simulink model "testBP"  (R2023a)
settings: Solver=VariableStepAuto  StartTime=0.0  StopTime=10.0  RelTol=1e-3
settings Model: Creator=grouleau  LastModifiedBy=grouleau
settings OptimizationCC: AccelVerboseBuild=on
settings SFSimCC: SimCustomHeaderCode="#include \"myFunc.h\""  SimUserSources=myFunc.c  SimDebugExecutionForCustomCode=on

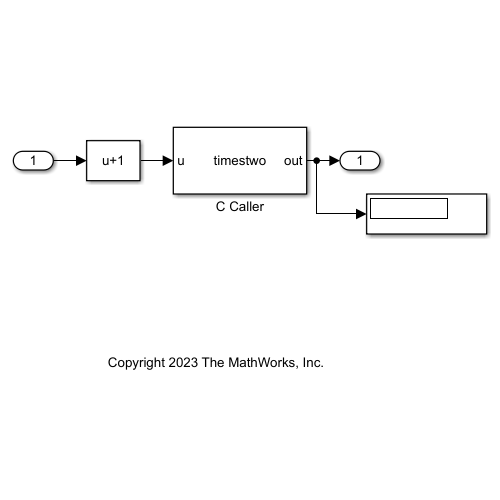
[thumbnail: Simulink's stored preview of the top-level diagram]
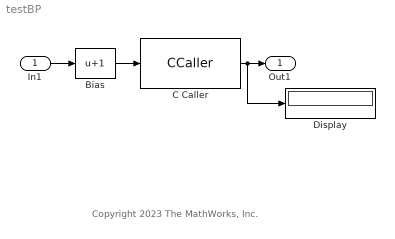
== system testBP ==
  note: Copyright 2023 The MathWorks, Inc.
  In1 : Inport  SampleTime=1
  Bias : Bias  Bias=1  SaturateOnIntegerOverflow=off
  C Caller : CCaller  FunctionName=timestwo  PortSpecificationStruct="%)30     .    N ,   8    (     @         %    \"     (    !     0         %  0 \"0    $    _    07)G3F%M90  4&]R=$YA;64 4V-O<&4     26YD97@     5'EP90      4VEZ90      27-';&]B86P   X    P    !@    @    $          4    (     0    ,    !         !   P!O=70 #@   #     &    \"     0         !0    @    !     P    $         $  # &]U=  .    .     8    (    !          %    \"     $    &     0         0    !@   $]U='!U=   #@   #@    &    \"     8         !0    @    !     0    $         \"0    @               X    X    !@    @    $          4    (     0    4    !         !     %    :6YT,S(    .    ,     8    (    !          %    \"     $    !     0         0  $ ,0    X    P    !@    @    ) @        4    (     0    $    !          (  0      #@   #     &    \"     0         !0    @    !     0    $         $  ! '4    .    ,     8    (    !          %    \"     $    !     0         0  $ =0    X    X    !@    @    $          4    (     0    4    !         !     %    26YP=70    .    .     8    (    !@         %    \"     $    !     0         )    \"               #@   #@    &    \"     0         !0    @    !    !0    $         $     4   !I;G0S,@    X    P    !@    @    $          4    (     0    $    !         !   0 Q    #@   #     &    \"     D\"        !0    @    !     0    $          @ !"
  Display : Display
  Out1 : Outport
  wires:
  In1/1 -> Bias/1
  Bias/1 -> C Caller/1
  C Caller/1 -> Display/1, Out1/1
